simulink model "senseo_model"  (R2018a)
settings: Solver=ode1  StartTime=0.0  StopTime=inf  FixedStep=1e-3  RelTol=1e-3
undefined symbols (not defined in the file or in its folder): ntc10k
libraries: fl_lib x24, nesl_utility x9, fluid x3, simulink x1, boiler x1, elec_lib x1, power_supply x1, pump x1
settings Model: Creator=ChLan  LastModifiedBy=ChLan
settings SimscapeCC: ExplicitSolverDiagnosticOptions=none  SimscapeLogType=all

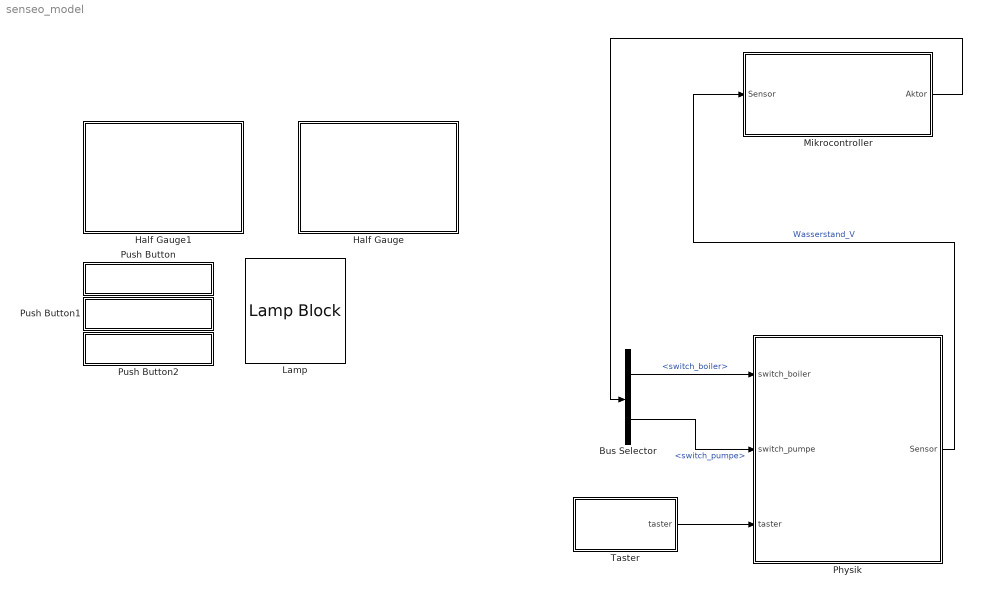
== system senseo_model ==
  Bus Selector : BusSelector  OutputSignals=switch_boiler,switch_pumpe
  Half Gauge : Subsystem  DialogController=hmiCreateDDGDialog  IsWebBlock=on  mask(MWDashboardBlock){webBlockId=947c324a-f2d6-4385-93d7-99386cc19ec6, webBlockType=semicirculargauge, ShowInLibBrowser=on, ShowInitialText=on, HMISrcModelName=senseo_model}
      mask prompts: webBlockId "WebBlock Id"; webBlockType "WebBlock Type"; HMISrcModelName "Source Model"
      mask help: SimulinkHMI:dialogs:SemicircularGaugeDialogDesc
      mask Help: helpview([docroot '/mapfiles/simulink.map'], 'hmi_half_gauge')
      mask Display:
      | if strcmp(get_param(bdroot(gcb),'BlockDiagramType'), 'library')
      |     image([(matlabroot) '/toolbox/simulink/hmi/icons/SemicircularGauge.png']);
      | end
  Half Gauge1 : Subsystem  DialogController=hmiCreateDDGDialog  IsWebBlock=on  mask(MWDashboardBlock){webBlockId=33aa71cf-ce5a-47cb-b958-916ba17b8f07, webBlockType=semicirculargauge, ShowInLibBrowser=on, ShowInitialText=on, HMISrcModelName=senseo_model}
      mask prompts: webBlockId "WebBlock Id"; webBlockType "WebBlock Type"; HMISrcModelName "Source Model"
      mask help: SimulinkHMI:dialogs:SemicircularGaugeDialogDesc
      mask Help: helpview([docroot '/mapfiles/simulink.map'], 'hmi_half_gauge')
      mask Display:
      | if strcmp(get_param(bdroot(gcb),'BlockDiagramType'), 'library')
      |     image([(matlabroot) '/toolbox/simulink/hmi/icons/SemicircularGauge.png']);
      | end
  Lamp : LampBlock  WebBlockId=478
  Mikrocontroller : Subsystem
  Physik : Subsystem
  Push Button : Subsystem  DialogController=hmiCreateDDGDialog  IsWebBlock=on  mask(MWDashboardBlock){webBlockId=77d0f651-8f95-4b89-b0d1-f4ff21e5f704, webBlockType=pushbutton, ShowInLibBrwoser=on, ShowInitialText=on, HMISrcModelName=senseo_model}
      mask prompts: webBlockId "WebBlock Id"; webBlockType "WebBlock Type"; HMISrcModelName "Source Model"
      mask help: SimulinkHMI:dialogs:PushButtonDialogDesc
      mask Help: helpview([docroot '/mapfiles/simulink.map'], 'hmi_push_button')
      mask Display:
      | model = bdroot(gcb);
      | if strcmp(get_param(model,'BlockDiagramType'), 'library')
      |     image([(matlabroot) '/toolbox/simulink/hmi/icons/PushButton.png']);
      | end
  Push Button1 : Subsystem  DialogController=hmiCreateDDGDialog  IsWebBlock=on  mask(MWDashboardBlock){webBlockId=8581b1ae-5f9d-4db0-b608-4b3498d1ee85, webBlockType=pushbutton, ShowInLibBrwoser=on, ShowInitialText=on, HMISrcModelName=senseo_model}
      mask prompts: webBlockId "WebBlock Id"; webBlockType "WebBlock Type"; HMISrcModelName "Source Model"
      mask help: SimulinkHMI:dialogs:PushButtonDialogDesc
      mask Help: helpview([docroot '/mapfiles/simulink.map'], 'hmi_push_button')
      mask Display:
      | model = bdroot(gcb);
      | if strcmp(get_param(model,'BlockDiagramType'), 'library')
      |     image([(matlabroot) '/toolbox/simulink/hmi/icons/PushButton.png']);
      | end
  Push Button2 : Subsystem  DialogController=hmiCreateDDGDialog  IsWebBlock=on  mask(MWDashboardBlock){webBlockId=35679551-ff79-47ee-bcc5-f967ea73a766, webBlockType=pushbutton, ShowInLibBrwoser=on, ShowInitialText=on, HMISrcModelName=senseo_model}
      mask prompts: webBlockId "WebBlock Id"; webBlockType "WebBlock Type"; HMISrcModelName "Source Model"
      mask help: SimulinkHMI:dialogs:PushButtonDialogDesc
      mask Help: helpview([docroot '/mapfiles/simulink.map'], 'hmi_push_button')
      mask Display:
      | model = bdroot(gcb);
      | if strcmp(get_param(model,'BlockDiagramType'), 'library')
      |     image([(matlabroot) '/toolbox/simulink/hmi/icons/PushButton.png']);
      | end
  Taster : Subsystem
  wires:
  Mikrocontroller/1(Aktor) -> Bus Selector/1
  Bus Selector/1 -> Physik/1(switch_boiler)  "<switch_boiler>"
  Bus Selector/2 -> Physik/2(switch_pumpe)  "<switch_pumpe>"
  Physik/1(Sensor) -> Mikrocontroller/1(Sensor)  "Wasserstand_V"
  Taster/1(taster) -> Physik/3(taster)

== system senseo_model/Half Gauge ==

== system senseo_model/Half Gauge1 ==

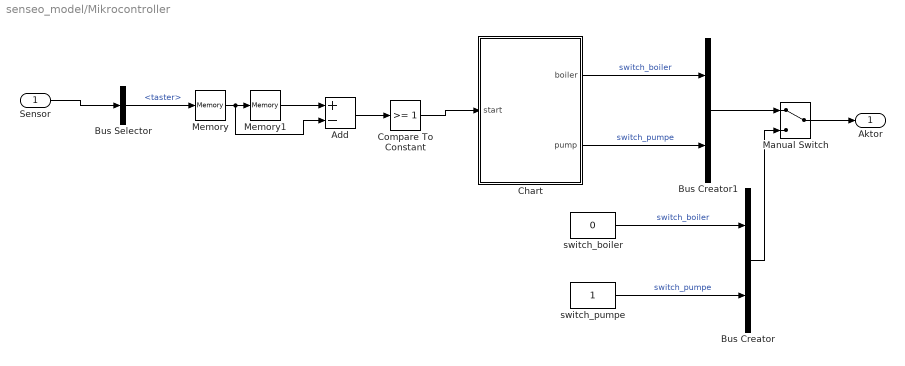
== system senseo_model/Mikrocontroller ==
  Sensor : Inport
  Add : Sum  Inputs=+-
  Bus Creator : BusCreator  Inputs=2
  Bus Creator1 : BusCreator  Inputs=2
  Bus Selector : BusSelector  OutputSignals=taster
  Chart : Stateflow chart  TreatAsAtomicUnit=on
  Compare To Constant : simulink/Logic and Bit Operations/Compare To Constant  relop=>=  const=1  OutDataTypeStr=boolean
  Manual Switch : ManualSwitch
  Memory : Memory
  Memory1 : Memory
  switch_boiler : Constant  Value=0
  switch_pumpe : Constant
  Aktor : Outport
  wires:
  switch_pumpe/1 -> Bus Creator/2  "switch_pumpe"
  switch_boiler/1 -> Bus Creator/1  "switch_boiler"
  Sensor/1 -> Bus Selector/1
  Bus Creator1/1 -> Manual Switch/1
  Chart/1(boiler) -> Bus Creator1/1  "switch_boiler"
  Chart/2(pump) -> Bus Creator1/2  "switch_pumpe"
  Bus Creator/1 -> Manual Switch/2
  Manual Switch/1 -> Aktor/1
  Bus Selector/1 -> Memory/1  "<taster>"
  Memory/1 -> Add/2, Memory1/1
  Memory1/1 -> Add/1
  Add/1 -> Compare To Constant/1
  Compare To Constant/1 -> Chart/1(start)

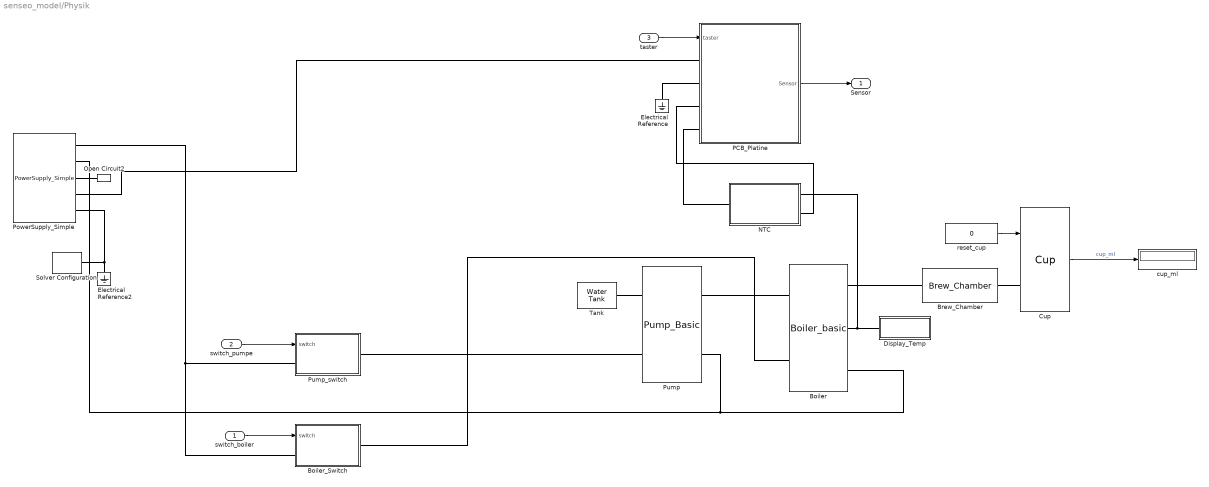
== system senseo_model/Physik ==
  switch_boiler : Inport
  switch_pumpe : Inport  Port=2
  taster : Inport  Port=3
  Boiler : boiler/Boiler_basic
  Boiler_Switch : Subsystem
  Brew_Chamber : fluid/Brew_Chamber
  Cup : fluid/Cup
  Display_Temp : Subsystem
  Electrical Reference : fl_lib/Electrical/Electrical Elements/Electrical Reference
  Electrical Reference2 : fl_lib/Electrical/Electrical Elements/Electrical Reference
  NTC : Subsystem  mask{res_table=ntc10k}
      mask prompts: res_table "T-R Table"
  Open Circuit2 : fl_lib/Electrical/Electrical Elements/Open Circuit  v_specify=off  v_priority=None  v=0 V  v_nominal_specify=off  v_nominal_unit=V  v_nominal_value=1
      settings: SourceProductName=Simscape  SourceProductBaseCode=SS
  PCB_Platine : Subsystem
  PowerSupply_Simple : power_supply/PowerSupply_Simple  VariantControl=1==1
  Pump : pump/Pump_Basic
  Pump_switch : Subsystem
  Solver Configuration : nesl_utility/Solver Configuration  PhysicalDomain=network_engine_domain  SubClassName=solver  LeftPortType=input  RightPortType=generic  Tones=[]  Harmonics=[]  SimulateNoise=off  Profile=off  UseLocalSampling=off  EnableSwitchedLinearOptims=on  FrequencyDomain=off  UseCCode=off  RelTol=0.001  AbsTol=1e-06  MinStep=1e-09  ToWorkspace=off  RevertToSquareIcSolve=off  NumHomotopyIterations=100  PhasorMode=off  PhasorModeNumHarmonics=1  DoDC=off  ResidualTolerance=1e-09  UseLocalSolver=off  LocalSolverChoice=NE_BACKWARD_EULER_ADVANCER  LocalSolverSampleTime=0.001  DoFixedCost=off  MaxNonlinIter=3  MaxModeIter=2  LinearAlgebra=Sparse  EquationFormulation=NE_TIME_EF  DelaysMemoryBudget=1024  AutomaticFiltering=on  FilteringTimeConstant=0.001
  Tank : fluid/Water Tank
  cup_ml : Display
  reset_cup : Constant  Value=0
  Sensor : Outport
  wires:
  switch_boiler/1 -> Boiler_Switch/1(switch)
  switch_pumpe/1 -> Pump_switch/1(switch)
  Cup/1 -> cup_ml/1  "cup_ml"
  reset_cup/1 -> Cup/1
  taster/1 -> PCB_Platine/1(taster)
  PCB_Platine/1(Sensor) -> Sensor/1
  connections:
  Pump/RConn1 -- Boiler/LConn1
  Pump/LConn1 -- Tank/LConn1
  Boiler_Switch/LConn1 -- PowerSupply_Simple/RConn1 -- Pump_switch/LConn1
  Brew_Chamber/LConn1 -- Boiler/RConn1
  Boiler_Switch/RConn1 -- Boiler/LConn2
  Electrical Reference2/LConn1 -- PowerSupply_Simple/RConn5 -- Solver Configuration/RConn1
  PowerSupply_Simple/RConn4 -- PCB_Platine/LConn1
  PowerSupply_Simple/RConn3 -- Open Circuit2/LConn1
  Pump/LConn2 -- Pump_switch/RConn1
  Boiler/RConn3 -- Pump/RConn2 -- PowerSupply_Simple/RConn2
  Boiler/RConn2 -- Display_Temp/LConn1 -- NTC/LConn1
  Cup/LConn1 -- Brew_Chamber/RConn1
  PCB_Platine/LConn2 -- Electrical Reference/LConn1
  PCB_Platine/LConn3 -- NTC/LConn2
  PCB_Platine/LConn4 -- NTC/RConn1

== system senseo_model/Push Button ==

== system senseo_model/Push Button1 ==

== system senseo_model/Push Button2 ==

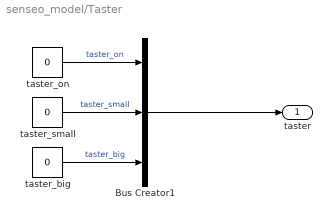
== system senseo_model/Taster ==
  Bus Creator1 : BusCreator  Inputs=3
  taster_big : Constant  Value=0
  taster_on : Constant  Value=0
  taster_small : Constant  Value=0
  taster : Outport
  wires:
  Bus Creator1/1 -> taster/1
  taster_big/1 -> Bus Creator1/3  "taster_big"
  taster_small/1 -> Bus Creator1/2  "taster_small"
  taster_on/1 -> Bus Creator1/1  "taster_on"

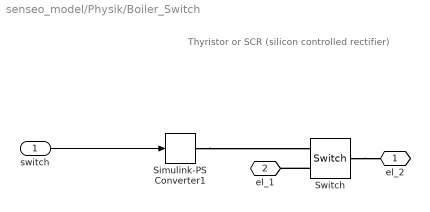
== system senseo_model/Physik/Boiler_Switch ==
  note: Thyristor or SCR (silicon controlled rectifier)
  switch : Inport
  Simulink-PS Converter1 : nesl_utility/Simulink-PS Converter  PhysicalDomain=network_engine_domain  SubClassName=ps_input  LeftPortType=input  RightPortType=output  PseudoPeriodic=off  Frequencies=[]  NoiseDistribution=none  NoiseParameters=[]  Unit=1  AffineConversion=off  FilteringAndDerivatives=provide  SimscapeFilterOrder=1  InputFilterTimeConstant=0.001  UdotUserProvided=0
  Switch : fl_lib/Electrical/Electrical Elements/Switch  R_closed=0.01 Ohm  G_open=1e-8 1/Ohm  Threshold=0  i_specify=off  i_priority=None  i=0 A  i_nominal_specify=off  i_nominal_unit=A  i_nominal_value=1  v_specify=off  v_priority=None  v=0 V  v_nominal_specify=off  v_nominal_unit=V  v_nominal_value=1
      settings: SourceProductName=Simscape
  el_2 : PMIOPort  Side=Left
  el_1 : PMIOPort  Port=2  Side=Right
  wires:
  switch/1 -> Simulink-PS Converter1/1
  connections:
  Simulink-PS Converter1/RConn1 -- Switch/RConn1
  Switch/RConn2 -- el_1/RConn1
  Switch/LConn1 -- el_2/RConn1

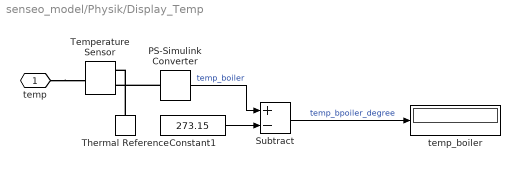
== system senseo_model/Physik/Display_Temp ==
  Constant1 : Constant  Value=273.15
  PS-Simulink Converter : nesl_utility/PS-Simulink Converter  PhysicalDomain=network_engine_domain  SubClassName=ps_output  LeftPortType=input  RightPortType=output  PseudoPeriodic=off  Frequencies=[]  Unit=1  AffineConversion=off
  Subtract : Sum  Inputs=+-
  Temperature Sensor : fl_lib/Thermal/Thermal Sensors/Temperature Sensor
  Thermal Reference : fl_lib/Thermal/Thermal Elements/Thermal Reference
  temp_boiler : Display
  temp : PMIOPort  Side=Left
  wires:
  PS-Simulink Converter/1 -> Subtract/1  "temp_boiler"
  Subtract/1 -> temp_boiler/1  "temp_bpoiler_degree"
  Constant1/1 -> Subtract/2
  connections:
  Thermal Reference/LConn1 -- Temperature Sensor/RConn1
  temp/RConn1 -- Temperature Sensor/LConn1
  PS-Simulink Converter/LConn1 -- Temperature Sensor/RConn2

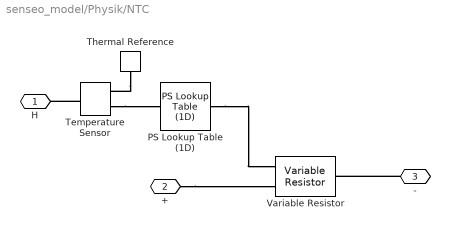
== system senseo_model/Physik/NTC ==
  PS Lookup Table (1D) : fl_lib/Physical Signals/Lookup Tables/PS Lookup Table (1D)  x=res_table(:,1) + 273.2  f=res_table(:,2)  interp_method=simscape.enum.interpolation.linear  extrap_method=simscape.enum.extrapolation.linear
      settings: SourceProductName=Simscape  SourceProductBaseCode=SS
  Temperature Sensor : fl_lib/Thermal/Thermal Sensors/Temperature Sensor
  Thermal Reference : fl_lib/Thermal/Thermal Elements/Thermal Reference
  Variable Resistor : fl_lib/Electrical/Electrical Elements/Variable Resistor  Rmin=0 Ohm  i_specify=off  i_priority=None  i=0 A  i_nominal_specify=off  i_nominal_unit=A  i_nominal_value=1  v_specify=off  v_priority=None  v=0 V  v_nominal_specify=off  v_nominal_unit=V  v_nominal_value=1
  H : PMIOPort  Side=Left
  + : PMIOPort  Port=2  Side=Left
  - : PMIOPort  Port=3  Side=Right
  connections:
  PS Lookup Table (1D)/RConn1 -- Variable Resistor/LConn1
  Temperature Sensor/RConn2 -- PS Lookup Table (1D)/LConn1
  +/RConn1 -- Variable Resistor/LConn2
  Temperature Sensor/LConn1 -- H/RConn1
  Thermal Reference/LConn1 -- Temperature Sensor/RConn1
  -/RConn1 -- Variable Resistor/RConn1

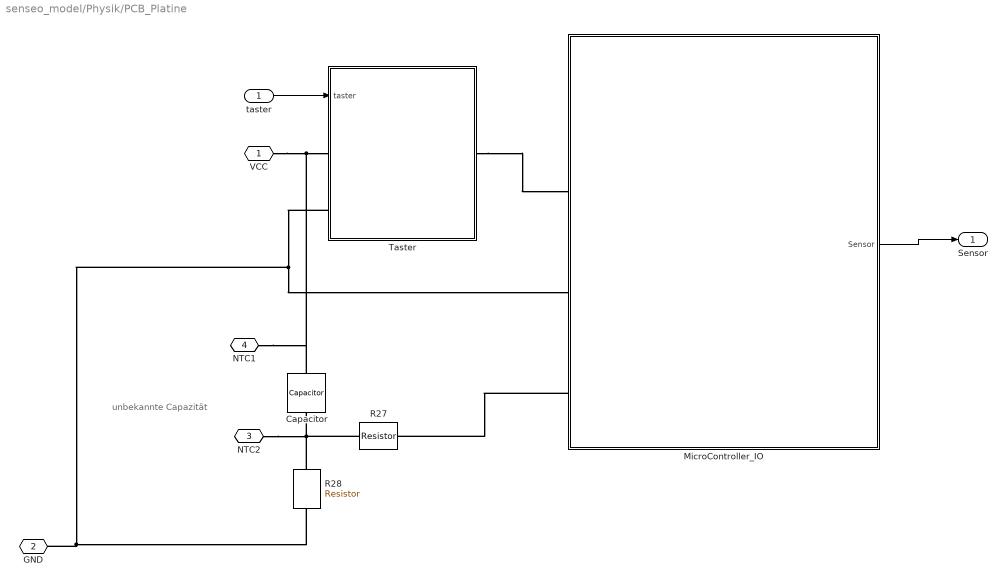
== system senseo_model/Physik/PCB_Platine ==
  note: unbekannte Capazität
  taster : Inport
  Capacitor : elec_lib/Passive Devices/Capacitor  enable_table=0  c=1e-6 F  Cvec=[1e-05, 1e-06] F  Vvec=[0, 10] V  CV_table_symmetry=1  C_tol=5  enable_C_tol=0  tol_distribution=1  nSigma=4  r=1e-6 Ohm  g=0 1/Ohm  enable_operating_limits=0  operating_limit_action=2  max_working_voltage_range=[-25, 25] V  power_rating=1 W  enable_faults=0  fault_action=1  Cscale_faulted=100  R_faulted=1e-3 Ohm  G_faulted=0 1/Ohm  tau_fault=1e-3 s  enable_temporal_fault=0  t_fault=1 s  enable_behavioral_fault=0  max_permissible_voltage_range=[-100, 100] V  t_fail_on_voltage=1 s  i_specify=off  i_priority=None  i=0 A  i_nominal_specify=off  i_nominal_unit=A  i_nominal_value=1  v_specify=off  v_priority=None  v=0 V  v_nominal_specify=off  v_nominal_unit=V  v_nominal_value=1  vc_specify=off  vc_priority=High  vc=0 V  vc_nominal_specify=off  vc_nominal_unit=V  vc_nominal_value=1
  MicroController_IO : Subsystem
  R27 : fl_lib/Electrical/Electrical Elements/Resistor  R=2.7 kOhm  i_specify=off  i_priority=None  i=0 A  i_nominal_specify=off  i_nominal_unit=A  i_nominal_value=1  v_specify=off  v_priority=None  v=0 V  v_nominal_specify=off  v_nominal_unit=V  v_nominal_value=1
      settings: AttributesFormatString=%<R> %<R_unit>
  R28 : fl_lib/Electrical/Electrical Elements/Resistor  R=1.8 kOhm  i_specify=off  i_priority=None  i=0 A  i_nominal_specify=off  i_nominal_unit=A  i_nominal_value=1  v_specify=off  v_priority=None  v=0 V  v_nominal_specify=off  v_nominal_unit=V  v_nominal_value=1
      settings: AttributesFormatString=%<R> %<R_unit>
  Taster : Subsystem
  VCC : PMIOPort  Side=Left
  GND : PMIOPort  Port=2  Side=Left
  NTC2 : PMIOPort  Port=3  Side=Left
  NTC1 : PMIOPort  Port=4  Side=Left
  Sensor : Outport
  wires:
  taster/1 -> Taster/1(taster)
  MicroController_IO/1(Sensor) -> Sensor/1
  connections:
  Taster/LConn2 -- MicroController_IO/LConn3 -- R28/RConn1 -- GND/RConn1
  VCC/RConn1 -- Taster/LConn1 -- NTC1/RConn1 -- Capacitor/LConn1
  Taster/RConn1 -- MicroController_IO/LConn2
  NTC2/RConn1 -- R27/LConn1 -- R28/LConn1 -- Capacitor/RConn1
  MicroController_IO/LConn4 -- R27/RConn1

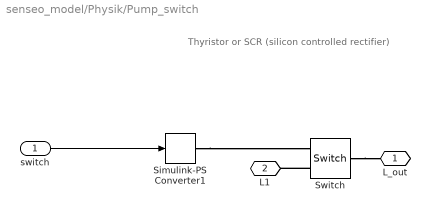
== system senseo_model/Physik/Pump_switch ==
  note: Thyristor or SCR (silicon controlled rectifier)
  switch : Inport
  Simulink-PS Converter1 : nesl_utility/Simulink-PS Converter  PhysicalDomain=network_engine_domain  SubClassName=ps_input  LeftPortType=input  RightPortType=output  PseudoPeriodic=off  Frequencies=[]  NoiseDistribution=none  NoiseParameters=[]  Unit=1  AffineConversion=off  FilteringAndDerivatives=provide  SimscapeFilterOrder=1  InputFilterTimeConstant=0.001  UdotUserProvided=0
  Switch : fl_lib/Electrical/Electrical Elements/Switch  R_closed=0.01 Ohm  G_open=1e-8 1/Ohm  Threshold=0  i_specify=off  i_priority=None  i=0 A  i_nominal_specify=off  i_nominal_unit=A  i_nominal_value=1  v_specify=off  v_priority=None  v=0 V  v_nominal_specify=off  v_nominal_unit=V  v_nominal_value=1
      settings: SourceProductName=Simscape
  L_out : PMIOPort  Side=Right
  L1 : PMIOPort  Port=2  Side=Left
  wires:
  switch/1 -> Simulink-PS Converter1/1
  connections:
  Simulink-PS Converter1/RConn1 -- Switch/RConn1
  Switch/RConn2 -- L1/RConn1
  Switch/LConn1 -- L_out/RConn1

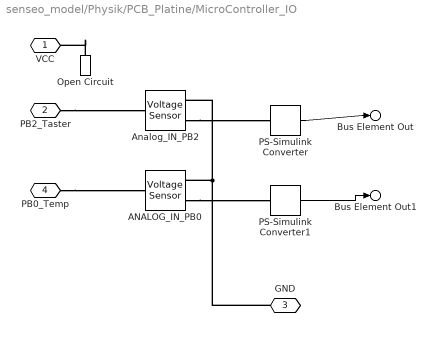
== system senseo_model/Physik/PCB_Platine/MicroController_IO ==
  ANALOG_IN_PB0 : fl_lib/Electrical/Electrical Sensors/Voltage Sensor
  Analog_IN_PB2 : fl_lib/Electrical/Electrical Sensors/Voltage Sensor
  Open Circuit : fl_lib/Electrical/Electrical Elements/Open Circuit  v_specify=off  v_priority=None  v=0 V  v_nominal_specify=off  v_nominal_unit=V  v_nominal_value=1
      settings: SourceProductName=Simscape  SourceProductBaseCode=SS
  PS-Simulink Converter : nesl_utility/PS-Simulink Converter  PhysicalDomain=network_engine_domain  SubClassName=ps_output  LeftPortType=input  RightPortType=output  PseudoPeriodic=off  Frequencies=[]  Unit=V  AffineConversion=off
  PS-Simulink Converter1 : nesl_utility/PS-Simulink Converter  PhysicalDomain=network_engine_domain  SubClassName=ps_output  LeftPortType=input  RightPortType=output  PseudoPeriodic=off  Frequencies=[]  Unit=V  AffineConversion=off
  VCC : PMIOPort  Side=Left
  PB2_Taster : PMIOPort  Port=2  Side=Left
  GND : PMIOPort  Port=3  Side=Left
  PB0_Temp : PMIOPort  Port=4  Side=Left
  Bus Element Out : Outport  PortName=Sensor  Element=taster
  Bus Element Out1 : Outport  PortName=Sensor  Element=temp
  wires:
  PS-Simulink Converter/1 -> Bus Element Out/1
  PS-Simulink Converter1/1 -> Bus Element Out1/1
  connections:
  PB2_Taster/RConn1 -- Analog_IN_PB2/LConn1
  GND/RConn1 -- ANALOG_IN_PB0/RConn2 -- Analog_IN_PB2/RConn2
  Analog_IN_PB2/RConn1 -- PS-Simulink Converter/LConn1
  Open Circuit/LConn1 -- VCC/RConn1
  ANALOG_IN_PB0/RConn1 -- PS-Simulink Converter1/LConn1
  PB0_Temp/RConn1 -- ANALOG_IN_PB0/LConn1

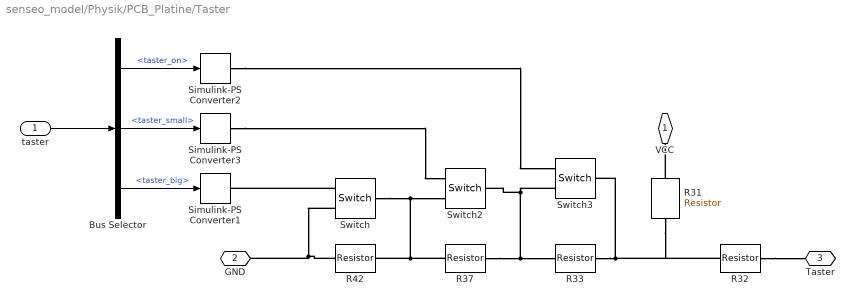
== system senseo_model/Physik/PCB_Platine/Taster ==
  taster : Inport
  Bus Selector : BusSelector  OutputSignals=taster_on,taster_small,taster_big
  R31 : fl_lib/Electrical/Electrical Elements/Resistor  R=12 kOhm  i_specify=off  i_priority=None  i=0 A  i_nominal_specify=off  i_nominal_unit=A  i_nominal_value=1  v_specify=off  v_priority=None  v=0 V  v_nominal_specify=off  v_nominal_unit=V  v_nominal_value=1
      settings: AttributesFormatString=%<R> %<R_unit>
  R32 : fl_lib/Electrical/Electrical Elements/Resistor  R=2.2 kOhm  i_specify=off  i_priority=None  i=0 A  i_nominal_specify=off  i_nominal_unit=A  i_nominal_value=1  v_specify=off  v_priority=None  v=0 V  v_nominal_specify=off  v_nominal_unit=V  v_nominal_value=1
      settings: AttributesFormatString=%<R> %<R_unit>
  R33 : fl_lib/Electrical/Electrical Elements/Resistor  R=12 kOhm  i_specify=off  i_priority=None  i=0 A  i_nominal_specify=off  i_nominal_unit=A  i_nominal_value=1  v_specify=off  v_priority=None  v=0 V  v_nominal_specify=off  v_nominal_unit=V  v_nominal_value=1
      settings: AttributesFormatString=%<R> %<R_unit>
  R37 : fl_lib/Electrical/Electrical Elements/Resistor  R=5.6 kOhm  i_specify=off  i_priority=None  i=0 A  i_nominal_specify=off  i_nominal_unit=A  i_nominal_value=1  v_specify=off  v_priority=None  v=0 V  v_nominal_specify=off  v_nominal_unit=V  v_nominal_value=1
      settings: AttributesFormatString=%<R> %<R_unit>
  R42 : fl_lib/Electrical/Electrical Elements/Resistor  R=2.7 kOhm  i_specify=off  i_priority=None  i=0 A  i_nominal_specify=off  i_nominal_unit=A  i_nominal_value=1  v_specify=off  v_priority=None  v=0 V  v_nominal_specify=off  v_nominal_unit=V  v_nominal_value=1
      settings: AttributesFormatString=%<R> %<R_unit>
  Simulink-PS Converter1 : nesl_utility/Simulink-PS Converter  PhysicalDomain=network_engine_domain  SubClassName=ps_input  LeftPortType=input  RightPortType=output  PseudoPeriodic=off  Frequencies=[]  NoiseDistribution=none  NoiseParameters=[]  Unit=1  AffineConversion=off  FilteringAndDerivatives=provide  SimscapeFilterOrder=1  InputFilterTimeConstant=0.001  UdotUserProvided=0
  Simulink-PS Converter2 : nesl_utility/Simulink-PS Converter  PhysicalDomain=network_engine_domain  SubClassName=ps_input  LeftPortType=input  RightPortType=output  PseudoPeriodic=off  Frequencies=[]  NoiseDistribution=none  NoiseParameters=[]  Unit=1  AffineConversion=off  FilteringAndDerivatives=provide  SimscapeFilterOrder=1  InputFilterTimeConstant=0.001  UdotUserProvided=0
  Simulink-PS Converter3 : nesl_utility/Simulink-PS Converter  PhysicalDomain=network_engine_domain  SubClassName=ps_input  LeftPortType=input  RightPortType=output  PseudoPeriodic=off  Frequencies=[]  NoiseDistribution=none  NoiseParameters=[]  Unit=1  AffineConversion=off  FilteringAndDerivatives=provide  SimscapeFilterOrder=1  InputFilterTimeConstant=0.001  UdotUserProvided=0
  Switch : fl_lib/Electrical/Electrical Elements/Switch  R_closed=0.01 Ohm  G_open=1e-8 1/Ohm  Threshold=0  i_specify=off  i_priority=None  i=0 A  i_nominal_specify=off  i_nominal_unit=A  i_nominal_value=1  v_specify=off  v_priority=None  v=0 V  v_nominal_specify=off  v_nominal_unit=V  v_nominal_value=1
      settings: SourceProductName=Simscape
  Switch2 : fl_lib/Electrical/Electrical Elements/Switch  R_closed=0.01 Ohm  G_open=1e-8 1/Ohm  Threshold=0  i_specify=off  i_priority=None  i=0 A  i_nominal_specify=off  i_nominal_unit=A  i_nominal_value=1  v_specify=off  v_priority=None  v=0 V  v_nominal_specify=off  v_nominal_unit=V  v_nominal_value=1
      settings: SourceProductName=Simscape
  Switch3 : fl_lib/Electrical/Electrical Elements/Switch  R_closed=0.01 Ohm  G_open=1e-8 1/Ohm  Threshold=0  i_specify=off  i_priority=None  i=0 A  i_nominal_specify=off  i_nominal_unit=A  i_nominal_value=1  v_specify=off  v_priority=None  v=0 V  v_nominal_specify=off  v_nominal_unit=V  v_nominal_value=1
      settings: SourceProductName=Simscape
  VCC : PMIOPort  Side=Left
  GND : PMIOPort  Port=2  Side=Left
  Taster : PMIOPort  Port=3  Side=Right
  wires:
  taster/1 -> Bus Selector/1
  Bus Selector/1 -> Simulink-PS Converter2/1  "<taster_on>"
  Bus Selector/2 -> Simulink-PS Converter3/1  "<taster_small>"
  Bus Selector/3 -> Simulink-PS Converter1/1  "<taster_big>"
  connections:
  Switch/RConn2 -- R42/LConn1 -- GND/RConn1
  R33/RConn1 -- R32/LConn1 -- R31/LConn1 -- Switch3/LConn1
  Switch/RConn1 -- Simulink-PS Converter1/RConn1
  Simulink-PS Converter2/RConn1 -- Switch3/RConn1
  R31/RConn1 -- VCC/RConn1
  Simulink-PS Converter3/RConn1 -- Switch2/RConn1
  R32/RConn1 -- Taster/RConn1
  R37/LConn1 -- Switch/LConn1 -- Switch2/RConn2 -- R42/RConn1
  R37/RConn1 -- R33/LConn1 -- Switch3/RConn2 -- Switch2/LConn1

== stateflow chart senseo_model/Mikrocontroller/Chart ==
  settings: updateMethod=DISCRETE
  state boot
  state off
  state heat_water
    boiler = 1
    pump = 0
  state brew
    boiler = 0
    pump = 1
  (default) -> boot
  boot -> off : after(0.1,sec)
  brew -> off : after(40,sec)
  off -> heat_water : [start]
  heat_water -> brew : after(40,sec)
  data: boiler output; pump output; start input
